simulink model "Dynamics_v2_temp"  (R2021b)
settings: Solver=VariableStepAuto  StartTime=0.0  StopTime=10.0  RelTol=1e-3
InitFcn:
  | % ************** Initiate forces
  | % f0=[0;0;0;0;0;0];
  | % f0=[0;0;0;0;0;0;0];
  | f_0=[0;0;0];
  | f_m=[0;0];
  | f_e=[0;0;0;0;0;0];
  | % ************** Initiate states
  | q_m=[0;0];
  | q_dot_m=[0;0];
  | P=[0;0;0];
  | V_I0=[0;0;0];
  | % ************** Load main
  | %run(Main.m)
values from neighbouring files (symbols this model uses):
  diag_M = diagonalize(M_frak0, M_frak)    [Internal_KUKA_Main.m]    (also in KUKA_Main.m; Main.m)
  g_bar = zeros(4,4,n)    [Internal_KUKA_Main.m]
  iota0 = eye(6,6)    [Internal_KUKA_Main.m]    (also in KUKA_Main.m; Main.m = [1 0 0; 0 1 0;zeros(3,3);0 0 1])
  M_curly = zeros(n,6,6)    [M_curly.m]    (also in M_curly_ee.m)
  mu = -10.*P0    [Initiate_FQ.m]    (also in Internal_KUKA_Main.m = P; KUKA_Main.m = P; Main.m = zeros(6,1)')
  Xi_m = Xi_m(1:robot.n*6,1:robot.n)    [Internal_KUKA_Main.m]    (also in KUKA_Main.m)
  Xi_m_matrix = zeros(6*n,n)    [Internal_KUKA_Main.m]    (also in KUKA_Main.m; Main.m)
undefined symbols (not defined in the file or in its folder): Ad_gm_inv, M_curly0
(part 2 of 2)

== matlab function Dynamics_v2_temp/Inverse Dynamics/Internal Dynamics/N_hat ==
  data: N_hat output; q_m input; q_dot_m input; Xi_m input; Xi_m_matrix input; M0 input; M0m input; A input; V_I0 input; P input; Lm input; Lm0 input
function N_hat = N_hat(q_m,q_dot_m,Xi_m,Xi_m_matrix, M0,M0m,A,V_I0,P,Lm,Lm0)
% Calculates the N_hat_m matrix from base pose and arm joint angles

n=length(q_m);

V=V_I0;

% Find Lm0
% for i=1:n
%     Lm0=Ad_frak(1,i,Xi_m,q_m);% equation 63 of TRO
% end

% Find partial of Lm0 to joint angles
Lm0_partial=zeros(6*n,6,n); % 6nx6xn
for i=1:n
    for j=1:n
        Lm0_partial(6*(j-1)+1:6*j,1:6,i)=Ad_partial(j,1,i,Xi_m,q_m); % equation 114 of TRO paper
    end
end

% Find partial of M0 to joint angles
M0_partial=zeros(6,6,n); %initiate
for i=1:n
    M0_partial(1:6,1:6,i)= transpose(Lm0_partial(i))*diagM*Lm0+transpose(Lm0)*diagM*Lm0_partial(i); %6x6 %equation 117 of TRO
end

% Find partial of M0m to joint angles
M0m_partial=zeros(6,n,n);
for i=1:n
    M0m_partial(6,n,i)= (transpose(Lm0_partial)*diagM*Lm0+transpose(Lm0)*diagM*Lm)*Xi_m_matrix; % equation 118 of TRO paper
end

% Find partial of connection A to each joint angle
A_partial=zeros(6,n,n);
for i=1:n
    A_partial(6,n,i)=inverse(M0)*M0_partial(1:6,1:6,i)*inverse(M0)*M0m+inverse(M0)*M0m_partial(6,n,i); % Equation 122
end


%Form N_hat from equation 19 of ACC paper
N_temp1=zeros(n,6); N_temp2=zeros(n,6); N_temp3=zeros(n,6);

for i=1:n
    N_temp1=N_temp1+transpose(A_partial(6,n,i).*q_dot_m(i)); % transpose of (6xn times 1x1)
    N_temp2(i,1:6)=transpose(q_dot_m)*transpose(A_partial(6,n,i)); %1xn times nx6
    N_temp3(i,1:6)=0.5*transpose(P)*M0_partial(1:6,1:6,i); % 1x6 times 6x6
end

N_hat=transpose(A)*transpose(adjoint_low(V))*P-N_temp1*P+N_temp2*P+N_temp3*P;

== matlab function Dynamics_v2_temp/time-dependent variables' calculations/  ==
  data: q_m input; L0 output; Lm0 output; Lm output; Xi_m input
function [L0,Lm0,Lm] =L_calculator(q_m,Xi_m)
% Calculates the time-dependent L matrix
n=length(q_m);
L=zeros(6*(n+1),6*(n+1));
% Compute M_frak for ith body
% Calculate L matrix
for i=1:n
    for j=1:n
        if i>j
            Ad_temp=eye(6);
            for k=i:j
                Ad_temp=Ad_temp*Adjoint(g_Matrix(-Xi_m(:,k),q_m(k)));
            end
            L(6*(i-1)+1:6*(i-1)+6,6*(j-1)+1:6*(j-1)+6)=Ad_temp;
        elseif i==j
            L(6*(i-1)+1:6*(i-1)+6,6*(j-1)+1:6*(j-1)+6)=eye(6);
        elseif i<j
            L(6*(i-1)+1:6*(i-1)+6,6*(j-1)+1:6*(j-1)+6)=zeros(6);
        end
    end
end

L0=L(1:6,1:6);
Lm0=L(7:end,1:6);
Lm=L(7:end,7:end);

end

== matlab function Dynamics_v2_temp/time-dependent variables' calculations/MATLAB Function ==
  data: M0 input; M0m input; A output
function A=A_connection(M0,M0m)
% Compute the connection A from mass properties

A=M0\M0m;

== matlab function Dynamics_v2_temp/time-dependent variables' calculations/Jacobian_ee ==
  data: J_e0 output; q_m input; Xi_m input; J_em output
function [J_e0, J_em] = Jacobian_end_effector(q_m,Xi_m)
% Calculates the body Velocity of end-effector from base pose and arm joint angles

% Compute the geometric Jacobian of the point rp
%   	rp  point of interest in inertial frame 
%       i   link number

n=length(q_m);

% Initiate
J=zeros(6,6 + n);
% Jm=zeros(6,robot.n);

% Vehicle portion
J0=eye(6,3);
J(1:6,1:6)=J0;

% ____________ Manipulator Jacobian _____________ %

% Initiate
j=1;
Jm=zeros(6,6+n);

Jm(1:6,j)=Xi_m(1:6,j);
for j=2:n %Iterate through all joints
    for i=1:j-1
        temp=Adjoint(g_Matrix(Xi_m(:,i),q_m(i)));
    end
    Jm(1:6,j)=temp*Xi_m(:,j);
end


J_ee0=[J0 Jm(1:6,1:n)];
% J_eeI=Adjoint(g_I0)*J_ee0; % transform to inertia

J_e0=J_ee0(1:6,1:3);
J_em=J_ee0(1:6,7:6+n);

end

== matlab function Dynamics_v2_temp/time-dependent variables' calculations/Mass Matrix Blocks/MATLAB Function ==
  data: diag_M input; m0_frak output; m_diag output
function [m0_frak,m_diag]=m_frak_decomp(diag_M)
% Compute the Mass Matrix of the multibody system.
%   Output:
%   M0      Spacecraft mass matrix 
%   M0m
%   Mm      Manipulator mass matrix

%n=length(q_m);

m0_frak=diag_M(1:6,1:6);
m_diag=diag_M(7:end,7:end);

== matlab function Dynamics_v2_temp/time-dependent variables' calculations/Mass Matrix Blocks/Mass_Matrix_Blocks1 ==
  data: m_diag input; Lm0 input; Lm input; Xi_m_matrix input; M0 output; M0m output; Mm output; iota0 input
function [M0,M0m,Mm]=Mass_Matrix(m_diag,Lm0,Lm,Xi_m_matrix,iota0)
% Compute the Mass Matrix of the multibody system.
%   Output:
%   M0      Spacecraft mass matrix 
%   M0m
%   Mm      Manipulator mass matrix

%n=length(q_m);

m0_frak=m_diag(1:6,1:6);
m_diag=m_diag(7:end,7:end);

%Initiate
M0=[I0,zeros(3,3);zeros(3,3),m0*eye(3)];
M0m=zeros(6,6*n);
Mm=zeros(6*n,6*n);

%calculate transposes
iota0T=transpose(iota0);
Lm0T=transpose(Lm0);
LmT=transpose(Lm);
Xi_mT=transpose(Xi_m_matrix);

% Vehicle Spacecraft Mass matrix block
M0=iota0T*(m0_frak+Lm0T*m_diag*Lm0)*iota0;

% Vehicle Spacecraft Mass matrix block
M0m=iota0T*Lm0T*m_diag*Lm*Xi_m_matrix;

% Vehicle Spacecraft Mass matrix block
Mm=Xi_mT*LmT*m_diag*Lm*Xi_m_matrix;



end

== matlab function Dynamics_v2_temp/Simulink Function12/MATLAB Function ==
  data: M_frak0 output; M_curly0 input; M_curly input; Ad_gm_inv input; M_frak output
function [M_frak0,M_frak] =M_frak(M_curly0,M_curly,Ad_gm_inv)
% Compute M_frak for ith body

M_frak0=M_curly0;
M_frak=zeros(length(squeeze(M_curly(:,1,1))),6,6);

% Calculate M_frak
for i=1:length(squeeze(M_curly(:,1,1)))
%     Adi_inv=inverse(Adjoint());
    M_frak(i,:,:)=transpose(Ad_gm_inv(:,:,i))*squeeze(M_curly(i,:,:))*Ad_gm_inv(:,:,i);
end

== matlab function Dynamics_v2_temp/time-dependent variables' calculations/V_I0 ==
  data: P input; A_connection input; q_dot_m input; M0 input; V_I0 output
function V_I0=V_I0(P,A_connection,q_dot_m,M0)
% Find the spaccecraft velocity V_I0
M0_inv=inv(M0);
% temp=P-transpose(A_connection)*q_dot_m;
V_I0=M0_inv\P-A_connection*q_dot_m;

== matlab function Dynamics_v2_temp/Differential Kinematics/MATLAB Function ==
  data: V_Ie output; q_dot_m input; J_e0 input; J_em input; V_I0 input
function V_Ie = Differential_Kinematics(q_dot_m, J_e0, J_em,  V_I0)
% Calculates the body Velocity of end-effector from base pose and arm joint angles
% Using equation 25 of ACC paper

% Calculate the mass matrix at this configuration
% [M0 M0m Mm]=Mass_Matrix(q_m);

% A_connection=inverse(M0)*M0m;

% Find V_I0 from the known total momentum and joint velocities
% V_I0=inverse(M0)*transpose(Adjoint(g_I0))*mu-A_connection*q_dot_m;

% Find the end effector boy velocity 
V_Ie=[J_e0 J_em]*[V_I0;q_dot_m];

== matlab function Dynamics_v2_temp/Simulink Function12/MATLAB Function1 ==
  data: M_frak0 input; M_frak input; diag_M output
function diag_M =diagonalize(M_frak0, M_frak)
% Compute M_frak for ith body
n=length(M_frak(:,1,1));

% Initiate
diag_M=zeros(6*(n+1),6*(n+1));

diag_M(1:6,1:6)=M_frak0;

% Calculate diag{M_frak}
for i=2:(n+1)
    diag_M(6*(i-1)+1:6*i,6*(i-1)+1:6*i)=M_frak(i-1,:,:);
end

end

== matlab function Dynamics_v2_temp/Simulink Function2/Mass_Matrix_Blocks1 ==
  data: I0 input; Im input; m0 input; mm input; M0 output; q_m input; M0m output; Mm output; Xi_m input
function [M0,M0m,Mm]=Mass_Matrix(I0,Im,m0,mm,q_m,Xi_m)
% Compute the Mass Matrix of the multibody system.
%   Output:
%   M0      Spacecraft mass matrix 
%   M0m
%   Mm      Manipulator mass matrix

n=length(q_m);

%Initiate
Mm=zeros(6,6,n,'like',I0);

% Calculate L matrix
for i=1:n
    for j=1:n
        if i>j
            Ad_temp=eye(6);
            for k=i:j
                Ad_temp=Ad_temp*Adjoint(g_matrix(-Xi_m(k),q_m(k)))
            end
            L(6*(i-1)+1:6*(i-1)+6,6*(j-1)+1:6*(j-1)+6)=Ad_temp;
        elseif i==j
            L(6*(i-1)+1:6*(i-1)+6,6*(j-1)+1:6*(j-1)+6)=zeros(6);
        elseif i<j
            L(6*(i-1)+1:6*(i-1)+6,6*(j-1)+1:6*(j-1)+6)=zeros(6);
        end
    end
end

%Backwards recursion
for i=n:-1:1
    %Initialize M 
    Mm(1:6,1:6,i)=[Im(1:3,1:3,i),zeros(3,3);zeros(3,3),mm(i)*eye(3)];
    for j=1:n-i
        Mm(1:6,1:6,i)=Mm_tilde(1:6,1:6,i)+Tij(1:6,1:6,i+j,i)'*Mm(1:6,1:6,i+j)*Tij(1:6,1:6,i+j,i);
        % Conjugation of the Inertia matrix by the translation matrix corresponding to CG
    end
end

% Spacecraft M tilde
M0=[I0,zeros(3,3);zeros(3,3),m0*eye(3)];
for j=1:n
    M0=M0+Ti0(1:6,1:6,j)'*Mm(1:6,1:6,j)*Ti0(1:6,1:6,j);
end


end

== matlab function Dynamics_v2_temp/Simulink Function/MATLAB Function ==
  data: g_I0 input; g_Ie output; q_m input; Xi_m input; g_bar input
function g_Ie = Forward_Kinematics(g_I0, q_m,Xi_m,g_bar)
% Calculates the absolute pose of end-effector from base pose and arm joint angles

% Initiate
g_Ie=g_I0; %the pose of the spacecraft

n=length(q_m);

for i=0:length(q_m)-1
    g_Ie=g_Ie*expm(skewsym(Xi_m(1:6,i))*q_m(i)); % the effect of the motion induced by each joint
end

g_Ie=g_Ie*g_bar(1:4,1:4,end); %multiply by the initial pose of the last link (wrist)

== matlab function Dynamics_v2_temp/Simulink Function2/Mass Matrix Blocks/MATLAB Function ==
  data: diag_M input; m0_frak output; m_diag output
function [m0_frak,m_diag]=m_frak_decomp(diag_M)
% Compute the Mass Matrix of the multibody system.
%   Output:
%   M0      Spacecraft mass matrix 
%   M0m
%   Mm      Manipulator mass matrix

%n=length(q_m);

m0_frak=diag_M(1:6,1:6);
m_diag=diag_M(7:end,7:end);

== matlab function Dynamics_v2_temp/Simulink Function3/MATLAB Function ==
  data: J_e0 output; q_m input; Xi_m input; J_em output
function [J_e0, J_em] = Jacobian_end_effector(q_m,Xi_m)
% Calculates the body Velocity of end-effector from base pose and arm joint angles

% Compute the geometric Jacobian of the point rp
%   	rp  point of interest in inertial frame 
%       i   link number

n=length(q_m);

% Initiate
J=zeros(6,6 + n);
% Jm=zeros(6,robot.n);

% Vehicle portion
J0=eye(6,6);
J(1:6,1:6)=J0;

% ____________ Manipulator Jacobian _____________ %

% Initiate
j=1;
Jm=zeros(6,6+n);

Jm(1:6,j)=Xi_m(1:6,j);
for j=2:n %Iterate through all joints
    for i=1:j-1
        temp=Adjoint(g_Matrix(Xi_m(:,i),q_m(i)));
    end
    Jm(1:6,j)=temp*Xi_m(:,j);
end


J_ee0=[J0 Jm(1:6,1:n)];
% J_eeI=Adjoint(g_I0)*J_ee0; % transform to inertia

J_e0=J_ee0(1:6,1:6);
J_em=J_ee0(1:6,7:6+n);

end
